simulink model "example_4DoF_SSC0511"  (R2021a)
settings: Solver=VariableStepAuto  StartTime=0.0  StopTime=100  MaxStep=1e-3  RelTol=1e-3
values from neighbouring files (symbols this model uses):
  Cf = 0.4*2*(Kf*m2f)^0.5    (= 1923.09929188)    [parameters.m]
  Cr = 0.4*2*(Kr*m2r)^0.5    (= 1980.32142573)    [parameters.m]
  Hp = 0.16    [parameters.m]
  Ip = 2000/2    (= 1000)    [parameters.m]
  Lf = m2r/m2*wb    (= 1.19956486486)    [parameters.m]
  Lr = m2f/m2*wb    (= 1.37043513514)    [parameters.m]
  m2 = m2f + m2r    (= 555)    [parameters.m]
libraries: fl_lib x49, nesl_utility x17, simulink x1
settings Model: Creator=hmiyagaw  LastModifiedBy=hmiyagaw
settings SimscapeCC: SimscapeLogType=all

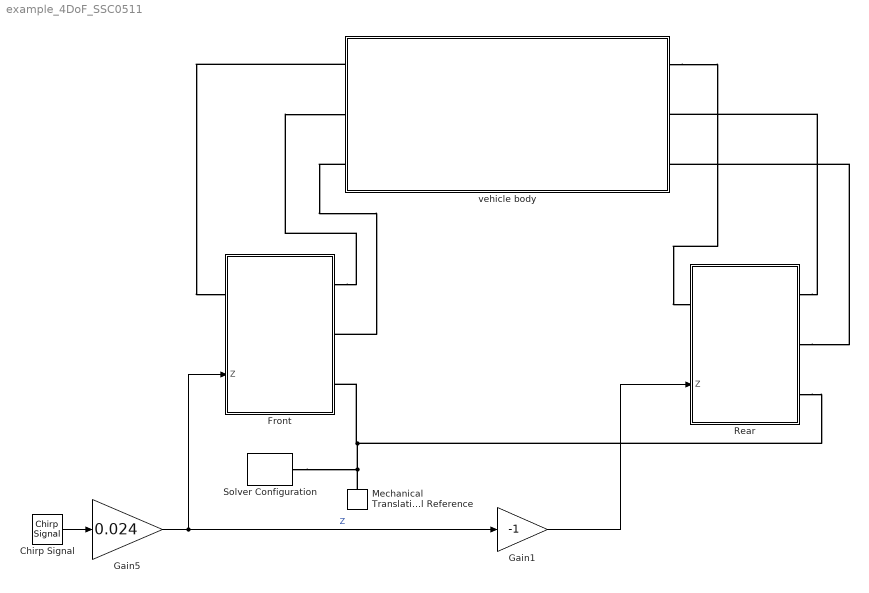
== system example_4DoF_SSC0511 ==
  Chirp Signal : simulink/Sources/Chirp Signal  f1=0  T=100  f2=10
  Front : Subsystem
      settings: PortSchema="{\"entries\":[{\"content\":{\"sides\":[{\"content\":{\"connectorIds\":[\"LConn1\",\"In1\"]},\"type\":\"ConnectorPlacement.EquallySpacedRectSide\",\"uuid\":\"3d63fa21-d947-4cf9-a1b1-7bf5a9f0119e\"},{\"content\":{\"connectorIds\":[\"RConn1\",\"RConn2\",\"RConn3\"],\"side\":\"RIGHT\"},\"type\":\"ConnectorPlacement.EquallySpacedRectSide\",\"uuid\":\"270d7113-fff1-4dd0-86df-3239146c0f37\"},{\"content\":{\"connectorIds\":[],\"side\":\"TOP\"},\"type\":\"ConnectorPlacement.EquallySpacedRectSide\",\"uuid\":\"96ae859e-a5bd-464f-a6dc-afd59e06ae9c\"}]},\"type\":\"ConnectorPlacement.EquallySpacedConnector\",\"uuid\":\"5116f963-09d4-4061-a830-9ee60a833058\"}],\"packageUris\":[\"http://schema.mathworks.com/mf0/Connector/R2020b\"],\"version\":\"1.0\"}"
  Gain1 : Gain  Gain=-1
  Gain5 : Gain  Gain=0.024
  Mechanical Translational Reference : fl_lib/Mechanical/Translational Elements/Mechanical Translational Reference
  Rear : Subsystem
      settings: PortSchema="{\"entries\":[{\"content\":{\"sides\":[{\"content\":{\"connectorIds\":[\"LConn1\",\"In1\"]},\"type\":\"ConnectorPlacement.EquallySpacedRectSide\",\"uuid\":\"3d63fa21-d947-4cf9-a1b1-7bf5a9f0119e\"},{\"content\":{\"connectorIds\":[\"RConn1\",\"RConn2\",\"RConn3\"],\"side\":\"RIGHT\"},\"type\":\"ConnectorPlacement.EquallySpacedRectSide\",\"uuid\":\"270d7113-fff1-4dd0-86df-3239146c0f37\"},{\"content\":{\"connectorIds\":[],\"side\":\"TOP\"},\"type\":\"ConnectorPlacement.EquallySpacedRectSide\",\"uuid\":\"96ae859e-a5bd-464f-a6dc-afd59e06ae9c\"}]},\"type\":\"ConnectorPlacement.EquallySpacedConnector\",\"uuid\":\"5116f963-09d4-4061-a830-9ee60a833058\"}],\"packageUris\":[\"http://schema.mathworks.com/mf0/Connector/R2020b\"],\"version\":\"1.0\"}"
  Solver Configuration : nesl_utility/Solver Configuration  PhysicalDomain=network_engine_domain  SubClassName=solver  LeftPortType=input  RightPortType=generic  Tones=[]  Harmonics=[]  SimulateNoise=off  Profile=off  UseLocalSampling=off  EnableSwitchedLinearOptims=on  FrequencyDomain=off  UseCCode=off  RelTol=0.001  AbsTol=1e-06  MinStep=1e-09  ToWorkspace=off  RevertToSquareIcSolve=off  NumHomotopyIterations=100  PhasorMode=off  PhasorModeNumHarmonics=1  DoDC=off  ResidualTolerance=1e-09  UseLocalSolver=off  LocalSolverChoice=NE_BACKWARD_EULER_ADVANCER  LocalSolverSampleTime=0.001  DoFixedCost=off  MaxNonlinIter=3  MaxModeIter=2  ComputeImpulses=off  ImpulseIterations=2  LinearAlgebra=auto  EquationFormulation=NE_TIME_EF  DelaysMemoryBudget=1024  AutomaticFiltering=on  FilteringTimeConstant=0.001  PartitionStorageMethod=AS_NEEDED  PartitionMemoryBudget=1024  PartitionMethod=ROBUST
      settings: SourceProductBaseCode=PW,SS
  vehicle body : Subsystem
  wires:
  Gain5/1 -> Front/1(Z), Gain1/1  "Z"
  Gain1/1 -> Rear/1(Z)
  Chirp Signal/1 -> Gain5/1
  connections:
  Mechanical Translational Reference/LConn1 -- Solver Configuration/RConn1 -- Rear/RConn3 -- Front/RConn3
  Front/RConn1 -- vehicle body/LConn2
  vehicle body/LConn1 -- Front/LConn1
  Rear/RConn1 -- vehicle body/RConn2
  vehicle body/RConn1 -- Rear/LConn1
  vehicle body/LConn3 -- Front/RConn2
  Rear/RConn2 -- vehicle body/RConn3

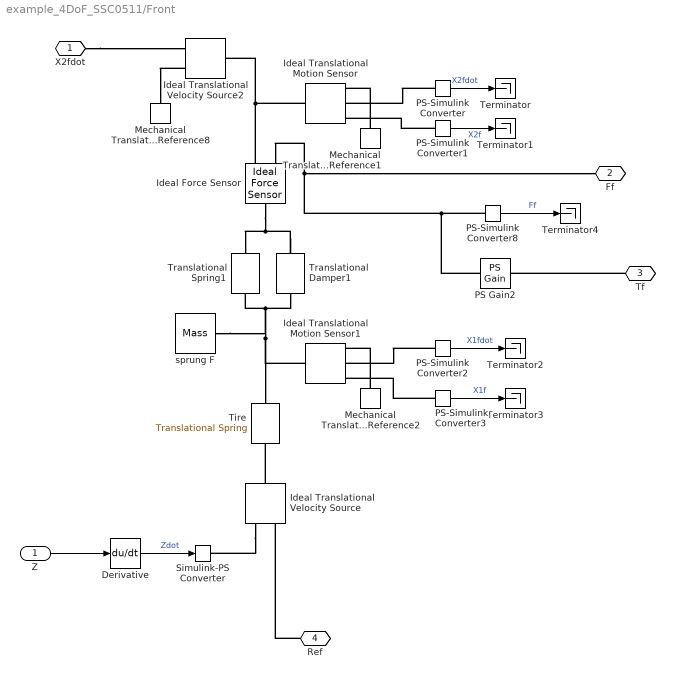
== system example_4DoF_SSC0511/Front ==
  Z : Inport
  Derivative : Derivative
  Ideal Force Sensor : fl_lib/Mechanical/Mechanical Sensors/Ideal Force Sensor
  Ideal Translational Motion Sensor : fl_lib/Mechanical/Mechanical Sensors/Ideal Translational Motion Sensor  offset=0 m
  Ideal Translational Motion Sensor1 : fl_lib/Mechanical/Mechanical Sensors/Ideal Translational Motion Sensor  offset=0 m
  Ideal Translational Velocity Source : fl_lib/Mechanical/Mechanical Sources/Ideal Translational Velocity Source
  Ideal Translational Velocity Source2 : fl_lib/Mechanical/Mechanical Sources/Ideal Translational Velocity Source
  Mechanical Translational Reference1 : fl_lib/Mechanical/Translational Elements/Mechanical Translational Reference
  Mechanical Translational Reference2 : fl_lib/Mechanical/Translational Elements/Mechanical Translational Reference
  Mechanical Translational Reference8 : fl_lib/Mechanical/Translational Elements/Mechanical Translational Reference
  PS Gain2 : fl_lib/Physical Signals/Functions/PS Gain  gain=-Lf m
      settings: AttributesFormatString=gain = %<gain>
  PS-Simulink Converter{,1..3,8} (5 alike) : nesl_utility/PS-Simulink Converter  PhysicalDomain=network_engine_domain  SubClassName=ps_output  LeftPortType=input  RightPortType=output  PseudoPeriodic=off  Frequencies=[]  Unit=1  AffineConversion=off
      settings: SourceProductBaseCode=PW,SS
  Simulink-PS Converter : nesl_utility/Simulink-PS Converter  PhysicalDomain=network_engine_domain  SubClassName=ps_input  LeftPortType=input  RightPortType=output  PseudoPeriodic=off  Frequencies=[]  NoiseDistribution=none  NoiseParameters=[]  Unit=1  AffineConversion=off  FilteringAndDerivatives=provide  SimscapeFilterOrder=1  InputFilterTimeConstant=0.001  UdotUserProvided=0
      settings: SourceProductBaseCode=PW,SS
  Terminator{,1..4} (5 alike) : Terminator
  Tire : fl_lib/Mechanical/Translational Elements/Translational Spring  spr_rate=Kt N/m  v_specify=off  v_priority=None  v=0 m/s  v_nominal_specify=off  v_nominal_unit=m/s  v_nominal_value=1  f_specify=off  f_priority=None  f=0 N  f_nominal_specify=off  f_nominal_unit=N  f_nominal_value=1  x_specify=on  x_priority=High  x=0 m  x_nominal_specify=off  x_nominal_unit=m  x_nominal_value=1
      settings: AttributesFormatString=spring rate = %<spr_rate>[N/m]
  Translational Damper1 : fl_lib/Mechanical/Translational Elements/Translational Damper  D=Cf N/(m/s)  v_specify=off  v_priority=None  v=0 m/s  v_nominal_specify=off  v_nominal_unit=m/s  v_nominal_value=1  f_specify=off  f_priority=None  f=0 N  f_nominal_specify=off  f_nominal_unit=N  f_nominal_value=1
      settings: AttributesFormatString=Damper Coef = %<D> %<D_unit>
  Translational Spring1 : fl_lib/Mechanical/Translational Elements/Translational Spring  spr_rate=Kf N/m  v_specify=off  v_priority=None  v=0 m/s  v_nominal_specify=off  v_nominal_unit=m/s  v_nominal_value=1  f_specify=off  f_priority=None  f=0 N  f_nominal_specify=off  f_nominal_unit=N  f_nominal_value=1  x_specify=off  x_priority=High  x=0 m  x_nominal_specify=off  x_nominal_unit=m  x_nominal_value=1
      settings: AttributesFormatString=spring rate = %<spr_rate>[N/m]
  sprung F : fl_lib/Mechanical/Translational Elements/Mass  mass=m1f kg  num_ports=foundation.enum.numPorts2.one  v_specify=off  v_priority=High  v=0 m/s  v_nominal_specify=off  v_nominal_unit=m/s  v_nominal_value=1  f_specify=off  f_priority=None  f=0 N  f_nominal_specify=off  f_nominal_unit=N  f_nominal_value=1
      settings: AttributesFormatString=mass = %<mass>[kg]
  X2fdot : PMIOPort  Side=Left
  Ff : PMIOPort  Port=2  Side=Right
  Tf : PMIOPort  Port=3  Side=Right
  Ref : PMIOPort  Port=4  Side=Right
  wires:
  Derivative/1 -> Simulink-PS Converter/1  "Zdot"
  PS-Simulink Converter/1 -> Terminator/1  "X2fdot"
  PS-Simulink Converter3/1 -> Terminator3/1  "X1f"
  PS-Simulink Converter2/1 -> Terminator2/1  "X1fdot"
  PS-Simulink Converter1/1 -> Terminator1/1  "X2f"
  Z/1 -> Derivative/1
  PS-Simulink Converter8/1 -> Terminator4/1  "Ff"
  connections:
  Ideal Translational Velocity Source/RConn1 -- Simulink-PS Converter/RConn1
  Translational Damper1/RConn1 -- Translational Spring1/RConn1 -- sprung F/LConn1 -- Ideal Translational Motion Sensor1/LConn1 -- Tire/LConn1
  Ideal Translational Motion Sensor/LConn1 -- Ideal Force Sensor/RConn1 -- Ideal Translational Velocity Source2/LConn1
  X2fdot/RConn1 -- Ideal Translational Velocity Source2/RConn1
  Translational Damper1/LConn1 -- Ideal Force Sensor/LConn1 -- Translational Spring1/LConn1
  Ideal Translational Velocity Source/LConn1 -- Tire/RConn1
  PS-Simulink Converter/LConn1 -- Ideal Translational Motion Sensor/RConn2
  Mechanical Translational Reference2/LConn1 -- Ideal Translational Motion Sensor1/RConn1
  PS-Simulink Converter2/LConn1 -- Ideal Translational Motion Sensor1/RConn2
  PS-Simulink Converter3/LConn1 -- Ideal Translational Motion Sensor1/RConn3
  PS-Simulink Converter1/LConn1 -- Ideal Translational Motion Sensor/RConn3
  Mechanical Translational Reference1/LConn1 -- Ideal Translational Motion Sensor/RConn1
  PS-Simulink Converter8/LConn1 -- Ff/RConn1 -- Ideal Force Sensor/RConn2 -- PS Gain2/LConn1
  Ideal Translational Velocity Source2/RConn2 -- Mechanical Translational Reference8/LConn1
  Ref/RConn1 -- Ideal Translational Velocity Source/RConn2
  Tf/RConn1 -- PS Gain2/RConn1

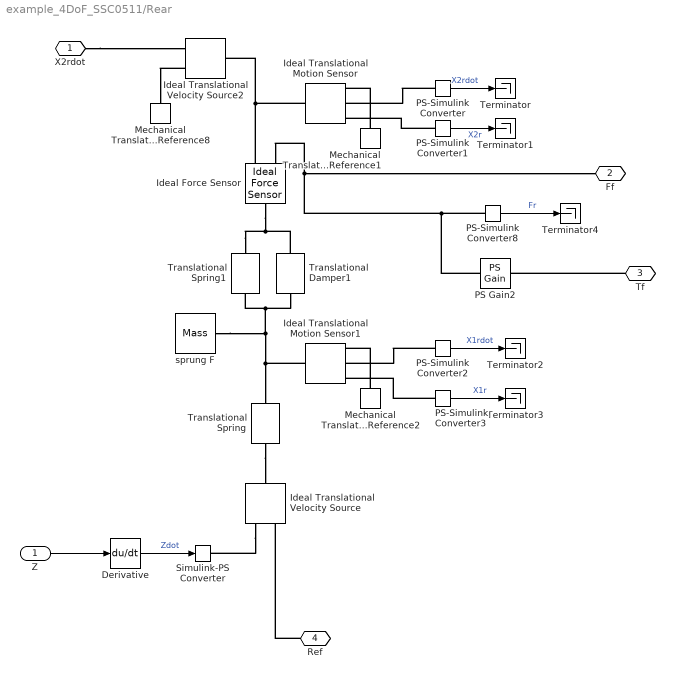
== system example_4DoF_SSC0511/Rear ==
  Z : Inport
  Derivative : Derivative
  Ideal Force Sensor : fl_lib/Mechanical/Mechanical Sensors/Ideal Force Sensor
  Ideal Translational Motion Sensor : fl_lib/Mechanical/Mechanical Sensors/Ideal Translational Motion Sensor  offset=0 m
  Ideal Translational Motion Sensor1 : fl_lib/Mechanical/Mechanical Sensors/Ideal Translational Motion Sensor  offset=0 m
  Ideal Translational Velocity Source : fl_lib/Mechanical/Mechanical Sources/Ideal Translational Velocity Source
  Ideal Translational Velocity Source2 : fl_lib/Mechanical/Mechanical Sources/Ideal Translational Velocity Source
  Mechanical Translational Reference1 : fl_lib/Mechanical/Translational Elements/Mechanical Translational Reference
  Mechanical Translational Reference2 : fl_lib/Mechanical/Translational Elements/Mechanical Translational Reference
  Mechanical Translational Reference8 : fl_lib/Mechanical/Translational Elements/Mechanical Translational Reference
  PS Gain2 : fl_lib/Physical Signals/Functions/PS Gain  gain=Lr m
      settings: AttributesFormatString=gain = %<gain>
  PS-Simulink Converter{,1..3,8} (5 alike) : nesl_utility/PS-Simulink Converter  PhysicalDomain=network_engine_domain  SubClassName=ps_output  LeftPortType=input  RightPortType=output  PseudoPeriodic=off  Frequencies=[]  Unit=1  AffineConversion=off
      settings: SourceProductBaseCode=PW,SS
  Simulink-PS Converter : nesl_utility/Simulink-PS Converter  PhysicalDomain=network_engine_domain  SubClassName=ps_input  LeftPortType=input  RightPortType=output  PseudoPeriodic=off  Frequencies=[]  NoiseDistribution=none  NoiseParameters=[]  Unit=1  AffineConversion=off  FilteringAndDerivatives=provide  SimscapeFilterOrder=1  InputFilterTimeConstant=0.001  UdotUserProvided=0
      settings: SourceProductBaseCode=PW,SS
  Terminator{,1..4} (5 alike) : Terminator
  Translational Damper1 : fl_lib/Mechanical/Translational Elements/Translational Damper  D=Cr N/(m/s)  v_specify=off  v_priority=None  v=0 m/s  v_nominal_specify=off  v_nominal_unit=m/s  v_nominal_value=1  f_specify=off  f_priority=None  f=0 N  f_nominal_specify=off  f_nominal_unit=N  f_nominal_value=1
      settings: AttributesFormatString=Damper Coef = %<D> %<D_unit>
  Translational Spring : fl_lib/Mechanical/Translational Elements/Translational Spring  spr_rate=Kt N/m  v_specify=off  v_priority=None  v=0 m/s  v_nominal_specify=off  v_nominal_unit=m/s  v_nominal_value=1  f_specify=off  f_priority=None  f=0 N  f_nominal_specify=off  f_nominal_unit=N  f_nominal_value=1  x_specify=on  x_priority=High  x=0 m  x_nominal_specify=off  x_nominal_unit=m  x_nominal_value=1
      settings: AttributesFormatString=spring rate = %<spr_rate>[N/m]
  Translational Spring1 : fl_lib/Mechanical/Translational Elements/Translational Spring  spr_rate=Kr N/m  v_specify=off  v_priority=None  v=0 m/s  v_nominal_specify=off  v_nominal_unit=m/s  v_nominal_value=1  f_specify=off  f_priority=None  f=0 N  f_nominal_specify=off  f_nominal_unit=N  f_nominal_value=1  x_specify=off  x_priority=High  x=0 m  x_nominal_specify=off  x_nominal_unit=m  x_nominal_value=1
      settings: AttributesFormatString=spring rate = %<spr_rate>[N/m]
  sprung F : fl_lib/Mechanical/Translational Elements/Mass  mass=m1r kg  num_ports=foundation.enum.numPorts2.one  v_specify=off  v_priority=High  v=0 m/s  v_nominal_specify=off  v_nominal_unit=m/s  v_nominal_value=1  f_specify=off  f_priority=None  f=0 N  f_nominal_specify=off  f_nominal_unit=N  f_nominal_value=1
      settings: AttributesFormatString=mass = %<mass>[kg]
  X2rdot : PMIOPort  Side=Left
  Ff : PMIOPort  Port=2  Side=Right
  Tf : PMIOPort  Port=3  Side=Right
  Ref : PMIOPort  Port=4  Side=Right
  wires:
  PS-Simulink Converter8/1 -> Terminator4/1  "Fr"
  Z/1 -> Derivative/1
  PS-Simulink Converter1/1 -> Terminator1/1  "X2r"
  PS-Simulink Converter2/1 -> Terminator2/1  "X1rdot"
  PS-Simulink Converter3/1 -> Terminator3/1  "X1r"
  PS-Simulink Converter/1 -> Terminator/1  "X2rdot"
  Derivative/1 -> Simulink-PS Converter/1  "Zdot"
  connections:
  Tf/RConn1 -- PS Gain2/RConn1
  Ref/RConn1 -- Ideal Translational Velocity Source/RConn2
  Ideal Translational Velocity Source2/RConn2 -- Mechanical Translational Reference8/LConn1
  PS Gain2/LConn1 -- PS-Simulink Converter8/LConn1 -- Ideal Force Sensor/RConn2 -- Ff/RConn1
  Mechanical Translational Reference1/LConn1 -- Ideal Translational Motion Sensor/RConn1
  PS-Simulink Converter1/LConn1 -- Ideal Translational Motion Sensor/RConn3
  PS-Simulink Converter3/LConn1 -- Ideal Translational Motion Sensor1/RConn3
  PS-Simulink Converter2/LConn1 -- Ideal Translational Motion Sensor1/RConn2
  Mechanical Translational Reference2/LConn1 -- Ideal Translational Motion Sensor1/RConn1
  PS-Simulink Converter/LConn1 -- Ideal Translational Motion Sensor/RConn2
  Translational Spring/RConn1 -- Ideal Translational Velocity Source/LConn1
  Translational Spring1/LConn1 -- Ideal Force Sensor/LConn1 -- Translational Damper1/LConn1
  X2rdot/RConn1 -- Ideal Translational Velocity Source2/RConn1
  Ideal Translational Velocity Source2/LConn1 -- Ideal Force Sensor/RConn1 -- Ideal Translational Motion Sensor/LConn1
  Translational Spring1/RConn1 -- Translational Spring/LConn1 -- Ideal Translational Motion Sensor1/LConn1 -- sprung F/LConn1 -- Translational Damper1/RConn1
  Ideal Translational Velocity Source/RConn1 -- Simulink-PS Converter/RConn1

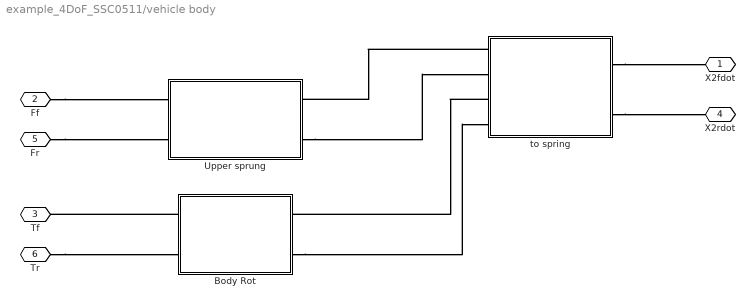
== system example_4DoF_SSC0511/vehicle body ==
  Body Rot : Subsystem
  Upper sprung : Subsystem
  to spring : Subsystem
  X2fdot : PMIOPort  Side=Left
  Ff : PMIOPort  Port=2  Side=Left
  Tf : PMIOPort  Port=3  Side=Left
  X2rdot : PMIOPort  Port=4  Side=Right
  Fr : PMIOPort  Port=5  Side=Right
  Tr : PMIOPort  Port=6  Side=Right
  connections:
  Ff/RConn1 -- Upper sprung/LConn1
  Tr/RConn1 -- Body Rot/LConn2
  to spring/LConn1 -- Upper sprung/RConn1
  to spring/LConn3 -- Body Rot/RConn1
  to spring/RConn1 -- X2fdot/RConn1
  Upper sprung/RConn2 -- to spring/LConn2
  Body Rot/RConn2 -- to spring/LConn4
  to spring/RConn2 -- X2rdot/RConn1
  Body Rot/LConn1 -- Tf/RConn1
  Fr/RConn1 -- Upper sprung/LConn2

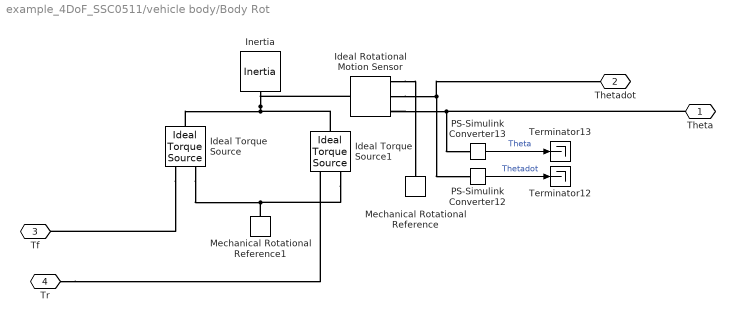
== system example_4DoF_SSC0511/vehicle body/Body Rot ==
  Ideal Rotational Motion Sensor : fl_lib/Mechanical/Mechanical Sensors/Ideal Rotational Motion Sensor  wrap_angle=simscape.enum.onoff.off  offset=0 rad
  Ideal Torque Source : fl_lib/Mechanical/Mechanical Sources/Ideal Torque Source
  Ideal Torque Source1 : fl_lib/Mechanical/Mechanical Sources/Ideal Torque Source
  Inertia : fl_lib/Mechanical/Rotational Elements/Inertia  inertia=m2*Hp^2 + Ip kg*m^2  num_ports=foundation.enum.numPorts2.one  w_specify=off  w_priority=High  w=0 rad/s  w_nominal_specify=off  w_nominal_unit=rad/s  w_nominal_value=1  t_specify=off  t_priority=None  t=0 N*m  t_nominal_specify=off  t_nominal_unit=N*m  t_nominal_value=1
      settings: AttributesFormatString=inertia = %<inertia>
  Mechanical Rotational Reference : fl_lib/Mechanical/Rotational Elements/Mechanical Rotational Reference
  Mechanical Rotational Reference1 : fl_lib/Mechanical/Rotational Elements/Mechanical Rotational Reference
  PS-Simulink Converter12 : nesl_utility/PS-Simulink Converter  PhysicalDomain=network_engine_domain  SubClassName=ps_output  LeftPortType=input  RightPortType=output  PseudoPeriodic=off  Frequencies=[]  Unit=1  AffineConversion=off
      settings: SourceProductBaseCode=PW,SS
  PS-Simulink Converter13 : nesl_utility/PS-Simulink Converter  PhysicalDomain=network_engine_domain  SubClassName=ps_output  LeftPortType=input  RightPortType=output  PseudoPeriodic=off  Frequencies=[]  Unit=1  AffineConversion=off
      settings: SourceProductBaseCode=PW,SS
  Terminator12 : Terminator
  Terminator13 : Terminator
  Theta : PMIOPort  Side=Right
  Thetadot : PMIOPort  Port=2  Side=Right
  Tf : PMIOPort  Port=3  Side=Left
  Tr : PMIOPort  Port=4  Side=Left
  wires:
  PS-Simulink Converter13/1 -> Terminator13/1  "Theta"
  PS-Simulink Converter12/1 -> Terminator12/1  "Thetadot"
  connections:
  Ideal Rotational Motion Sensor/RConn1 -- Mechanical Rotational Reference/LConn1
  Ideal Torque Source/RConn1 -- Tf/RConn1
  Inertia/LConn1 -- Ideal Rotational Motion Sensor/LConn1 -- Ideal Torque Source1/LConn1 -- Ideal Torque Source/LConn1
  Mechanical Rotational Reference1/LConn1 -- Ideal Torque Source1/RConn2 -- Ideal Torque Source/RConn2
  Tr/RConn1 -- Ideal Torque Source1/RConn1
  Ideal Rotational Motion Sensor/RConn3 -- PS-Simulink Converter13/LConn1 -- Theta/RConn1
  Ideal Rotational Motion Sensor/RConn2 -- Thetadot/RConn1 -- PS-Simulink Converter12/LConn1

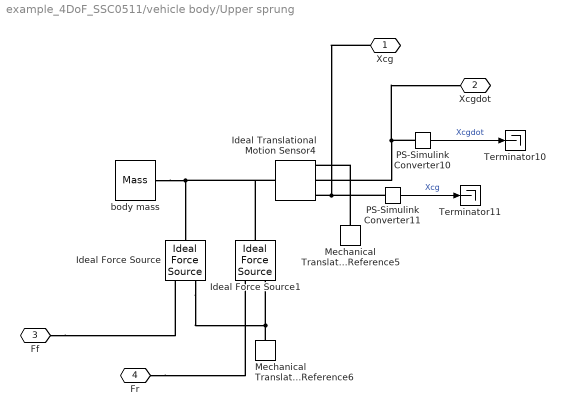
== system example_4DoF_SSC0511/vehicle body/Upper sprung ==
  Ideal Force Source : fl_lib/Mechanical/Mechanical Sources/Ideal Force Source
  Ideal Force Source1 : fl_lib/Mechanical/Mechanical Sources/Ideal Force Source
  Ideal Translational Motion Sensor4 : fl_lib/Mechanical/Mechanical Sensors/Ideal Translational Motion Sensor  offset=0 m
  Mechanical Translational Reference5 : fl_lib/Mechanical/Translational Elements/Mechanical Translational Reference
  Mechanical Translational Reference6 : fl_lib/Mechanical/Translational Elements/Mechanical Translational Reference
  PS-Simulink Converter10 : nesl_utility/PS-Simulink Converter  PhysicalDomain=network_engine_domain  SubClassName=ps_output  LeftPortType=input  RightPortType=output  PseudoPeriodic=off  Frequencies=[]  Unit=1  AffineConversion=off
      settings: SourceProductBaseCode=PW,SS
  PS-Simulink Converter11 : nesl_utility/PS-Simulink Converter  PhysicalDomain=network_engine_domain  SubClassName=ps_output  LeftPortType=input  RightPortType=output  PseudoPeriodic=off  Frequencies=[]  Unit=1  AffineConversion=off
      settings: SourceProductBaseCode=PW,SS
  Terminator10 : Terminator
  Terminator11 : Terminator
  body mass : fl_lib/Mechanical/Translational Elements/Mass  mass=m2 kg  num_ports=foundation.enum.numPorts2.one  v_specify=off  v_priority=High  v=0 m/s  v_nominal_specify=off  v_nominal_unit=m/s  v_nominal_value=1  f_specify=off  f_priority=None  f=0 N  f_nominal_specify=off  f_nominal_unit=N  f_nominal_value=1
      settings: AttributesFormatString=mass = %<mass>[kg]
  Xcg : PMIOPort  Side=Right
  Xcgdot : PMIOPort  Port=2  Side=Right
  Ff : PMIOPort  Port=3  Side=Left
  Fr : PMIOPort  Port=4  Side=Left
  wires:
  PS-Simulink Converter10/1 -> Terminator10/1  "Xcgdot"
  PS-Simulink Converter11/1 -> Terminator11/1  "Xcg"
  connections:
  Fr/RConn1 -- Ideal Force Source1/RConn1
  body mass/LConn1 -- Ideal Force Source1/LConn1 -- Ideal Translational Motion Sensor4/LConn1 -- Ideal Force Source/LConn1
  PS-Simulink Converter11/LConn1 -- Xcg/RConn1 -- Ideal Translational Motion Sensor4/RConn3
  Mechanical Translational Reference6/LConn1 -- Ideal Force Source1/RConn2 -- Ideal Force Source/RConn2
  Mechanical Translational Reference5/LConn1 -- Ideal Translational Motion Sensor4/RConn1
  PS-Simulink Converter10/LConn1 -- Ideal Translational Motion Sensor4/RConn2 -- Xcgdot/RConn1
  Ff/RConn1 -- Ideal Force Source/RConn1

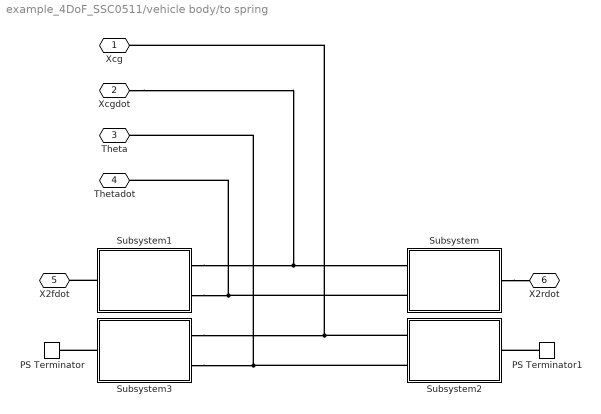
== system example_4DoF_SSC0511/vehicle body/to spring ==
  PS Terminator : fl_lib/Physical Signals/Sinks/PS Terminator
  PS Terminator1 : fl_lib/Physical Signals/Sinks/PS Terminator
  Subsystem : Subsystem
  Subsystem1 : Subsystem
  Subsystem2 : Subsystem
  Subsystem3 : Subsystem
  Xcg : PMIOPort  Side=Left
  Xcgdot : PMIOPort  Port=2  Side=Left
  Theta : PMIOPort  Port=3  Side=Left
  Thetadot : PMIOPort  Port=4  Side=Left
  X2fdot : PMIOPort  Port=5  Side=Right
  X2rdot : PMIOPort  Port=6  Side=Right
  connections:
  Subsystem2/LConn2 -- Subsystem3/LConn2 -- Theta/RConn1
  Subsystem/RConn1 -- X2rdot/RConn1
  Subsystem2/LConn1 -- Subsystem3/LConn1 -- Xcg/RConn1
  Subsystem1/RConn1 -- X2fdot/RConn1
  PS Terminator1/LConn1 -- Subsystem2/RConn1
  Subsystem/LConn2 -- Subsystem1/LConn2 -- Thetadot/RConn1
  Subsystem1/LConn1 -- Subsystem/LConn1 -- Xcgdot/RConn1
  Subsystem3/RConn1 -- PS Terminator/LConn1

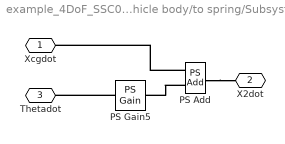
== system example_4DoF_SSC0511/vehicle body/to spring/Subsystem ==
  PS Add : fl_lib/Physical Signals/Functions/PS Add
  PS Gain5 : fl_lib/Physical Signals/Functions/PS Gain  gain=Lr m
      settings: AttributesFormatString=gain = %<gain>
  Xcgdot : PMIOPort  Side=Left
  X2dot : PMIOPort  Port=2  Side=Right
  Thetadot : PMIOPort  Port=3  Side=Left
  connections:
  PS Add/RConn1 -- X2dot/RConn1
  PS Gain5/LConn1 -- Thetadot/RConn1
  PS Add/LConn2 -- PS Gain5/RConn1
  PS Add/LConn1 -- Xcgdot/RConn1

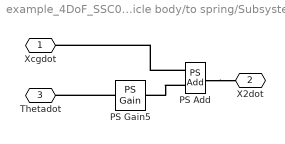
== system example_4DoF_SSC0511/vehicle body/to spring/Subsystem1 ==
  PS Add : fl_lib/Physical Signals/Functions/PS Add
  PS Gain5 : fl_lib/Physical Signals/Functions/PS Gain  gain=-Lf m
      settings: AttributesFormatString=gain = %<gain>
  Xcgdot : PMIOPort  Side=Left
  X2dot : PMIOPort  Port=2  Side=Right
  Thetadot : PMIOPort  Port=3  Side=Left
  connections:
  PS Add/LConn1 -- Xcgdot/RConn1
  PS Add/LConn2 -- PS Gain5/RConn1
  PS Gain5/LConn1 -- Thetadot/RConn1
  PS Add/RConn1 -- X2dot/RConn1

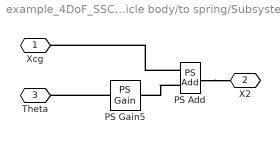
== system example_4DoF_SSC0511/vehicle body/to spring/Subsystem2 ==
  PS Add : fl_lib/Physical Signals/Functions/PS Add
  PS Gain5 : fl_lib/Physical Signals/Functions/PS Gain  gain=Lr m
      settings: AttributesFormatString=gain = %<gain>
  Xcg : PMIOPort  Side=Left
  X2 : PMIOPort  Port=2  Side=Right
  Theta : PMIOPort  Port=3  Side=Left
  connections:
  PS Add/LConn1 -- Xcg/RConn1
  PS Add/LConn2 -- PS Gain5/RConn1
  PS Gain5/LConn1 -- Theta/RConn1
  PS Add/RConn1 -- X2/RConn1

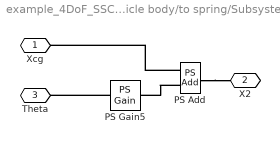
== system example_4DoF_SSC0511/vehicle body/to spring/Subsystem3 ==
  PS Add : fl_lib/Physical Signals/Functions/PS Add
  PS Gain5 : fl_lib/Physical Signals/Functions/PS Gain  gain=-Lf m
      settings: AttributesFormatString=gain = %<gain>
  Xcg : PMIOPort  Side=Left
  X2 : PMIOPort  Port=2  Side=Right
  Theta : PMIOPort  Port=3  Side=Left
  connections:
  PS Add/RConn1 -- X2/RConn1
  PS Gain5/LConn1 -- Theta/RConn1
  PS Add/LConn2 -- PS Gain5/RConn1
  PS Add/LConn1 -- Xcg/RConn1
